simulink model "xytheta_microcontroller"  (R2022a)
settings: Solver=VariableStepAuto  StartTime=0.0  StopTime=stop_time  RelTol=1e-3
values from neighbouring files (symbols this model uses):
  a1 = [0.0226481432906 0.0228584411445 0.0225295964484 0.0217518027828 0.0203868263557 0.0184221135046 0.0156410240283 0.0121230277389 0.00798950755081 0.00344770073943 -0.00140524350521 -0.00605971322152 ... (2997 elements, 37x9x9)]    [femm_output.mat]    (also in hi.mat = [0.040259405186 0.0403013496491 0.0403539168343 0.0403184727; test.mat = [0.0334886294169 0.0187353722544 -0.0188188604787 -0.0334886)
  a2 = [0.0289816801878 0.0282562064819 0.0268804805083 0.0249372347426 0.0221345937075 0.0184340302923 0.0137477378532 0.00803353156156 0.0017047126462 -0.0048350371899 -0.0110157154995 -0.01647453575 ... (2997 elements, 37x9x9)]    [femm_output.mat]    (also in hi.mat = [0.0510882717013 0.051015840912 0.0508647790068 0.0507223197; test.mat = [0.0338593341727 0.0189905412856 -0.0197522315336 -0.0338593)
  a3 = [0.0115535270098 0.0148029062382 0.0173877315644 0.0193612077509 0.0206442979737 0.0215000532697 0.021876503755 0.0217878376451 0.0212671436174 0.0202424961232 0.0185927416037 0.0163372080044 ... (2997 elements, 37x9x9)]    [femm_output.mat]    (also in hi.mat = [0.0214255858237 0.0226377892342 0.0238084550149 0.024930652; test.mat = [0.0190432080829 0.0343100490551 0.0190529625979 -0.01904320)
  a4 = [0.0199201516492 0.0239463634306 0.0268101507336 0.0287527989045 0.0300172301517 0.0306310326126 0.0306116684575 0.0301535034256 0.0292209899207 0.0275296444333 0.0250546319784 0.0217006548338 ... (2997 elements, 37x9x9)]    [femm_output.mat]    (also in hi.mat = [0.0351552019156 0.0366796893809 0.0381457834123 0.039508739; test.mat = [0.0191793003104 0.0345170149993 0.0192239303836 -0.01917930)
  b1 = [-0.0198768129153 -0.0149244319576 -0.00858526905599 -0.00187364461528 0.0050977168348 0.0114478894775 0.0171037743603 0.0216638634405 0.0251231705896 0.0275944419023 0.0292021825363 0.0301941032583 ... (2997 elements, 37x9x9)]    [femm_output.mat]    (also in hi.mat = [-0.0351292809325 -0.0335210392107 -0.0318149846307 -0.03001; test.mat = [-0.0195035950206 0.0204454837762 0.032908216348 0.019503595)
  b2 = [-0.0115479896023 -0.00770288201737 -0.00341093185035 0.0012077259201 0.00577057398931 0.00982413393911 0.0134313300768 0.0163555375406 0.0185311126654 0.0202513667265 0.0212470983786 0.0217997189875 ... (2997 elements, 37x9x9)]    [femm_output.mat]    (also in hi.mat = [-0.0214309796469 -0.0201513971109 -0.018842107593 -0.017472; test.mat = [-0.0191855417866 0.0192130384034 0.0341712245421 0.01918554)
  b3 = [-0.0290438679046 -0.0293208138251 -0.0289621611228 -0.0282127308736 -0.0266510102895 -0.0242723997603 -0.0209097969042 -0.0164709315768 -0.011084328795 -0.00477482143157 0.00165462601804 0.00800924150907 ... (2997 elements, 37x9x9)]    [femm_output.mat]    (also in hi.mat = [-0.0511327637629 -0.0511785516059 -0.0512008658749 -0.05117; test.mat = [-0.0346544389103 -0.0187806132998 0.0188182643543 0.0346544)
  b4 = [-0.0226529885689 -0.0220487060527 -0.0209138863789 -0.0192567684963 -0.016982348983 -0.0139643562445 -0.0103025939746 -0.00604882885267 -0.00143455513257 0.00343618932918 0.00801414292928 0.012190086562 ... (2997 elements, 37x9x9)]    [femm_output.mat]    (also in hi.mat = [-0.0402522375725 -0.0401755201934 -0.0400474470218 -0.03988; test.mat = [-0.033778561725 -0.0189587155081 0.0201521885325 0.03377856)
  c1 = [-0.018042933605 -0.0207358233247 -0.0226807589747 -0.0238865774927 -0.0245474910314 -0.0246583171435 -0.0242673887984 -0.0234585855422 -0.0221202260013 -0.0200782518148 -0.017518348181 -0.0141731707546 ... (2997 elements, 37x9x9)]    [femm_output.mat]    (also in hi.mat = [-0.0297253197394 -0.0308627231265 -0.0319523431791 -0.03294; test.mat = [-0.0182900065298 -0.0340093058074 -0.0190263778387 0.018290)
  c2 = [-0.0111046794327 -0.0156541395447 -0.0193854693358 -0.0221379319248 -0.0242137197455 -0.0256527501849 -0.0265983628578 -0.0270163619409 -0.0268882455917 -0.0262763125893 -0.0249792360852 -0.0229784347415 ... (2997 elements, 37x9x9)]    [femm_output.mat]    (also in hi.mat = [-0.0234193013701 -0.0250617295759 -0.0266424676889 -0.02819; test.mat = [-0.0188563417261 -0.033847126142 -0.0190525067235 0.0188563)
  c3 = [0.0110989874251 0.00587027765918 4.48039996108e-05 -0.00583886766056 -0.0113087799728 -0.0160948615017 -0.0199647800731 -0.0229326844268 -0.0249385554175 -0.0262624574827 -0.0268970230309 -0.0270019496976 ... (2997 elements, 37x9x9)]    [femm_output.mat]    (also in hi.mat = [0.0233910963939 0.0216737015426 0.0198604309257 0.018009200; test.mat = [0.0190983781671 -0.0185938316594 -0.0330743417046 -0.019098)
  c4 = [0.0180276596334 0.0143851403822 0.0100683328735 0.00515693164411 -8.40566002638e-05 -0.00533297487089 -0.0100594562482 -0.0142052505478 -0.017542507454 -0.0201282699008 -0.0221308552047 -0.0234805966963 ... (2997 elements, 37x9x9)]    [femm_output.mat]    (also in hi.mat = [0.0297436396273 0.0285474856426 0.0272933586912 0.025981890; test.mat = [0.0190714466776 -0.0196627612069 -0.0337734384564 -0.019071)
  theta_r_in = [0 5 10 15 20 25 30 35 40 45 50 55 ... (37 elements, 1x37)]    [femm_output.mat]    (also in hi.mat = [0 1 2 3 4 5 6 7 8 9 10 11 ... (180 elements, 1x180)]; test.mat = [0 30 60 90 120 150])
  x_position = [-2 -1.5 -1 -0.5 0 0.5 1 1.5 2]    [femm_output.mat]    (also in hi.mat; test.mat = 0)
  y_position = [-2 -1.5 -1 -0.5 0 0.5 1 1.5 2]    [femm_output.mat]    (also in hi.mat; test.mat = 0)
undefined symbols (not defined in the file or in its folder): fs_theta, x_sampletime, y_sampletime
libraries: dspsrcs4 x3, simulink x1
settings Model: Creator=qorgud1209  LastModifiedBy=baikhyeongmeon
settings DebuggingCC: UnconnectedInputMsg=warning  UnconnectedOutputMsg=warning  UnconnectedLineMsg=warning
settings SFSimCC: SimCustomHeaderCode="#include \"microcontroller.h\""  SimUserSources=microcontroller.c  SimAnalyzeCustomCode=on  CustomCodeGlobalsAsFunctionIO=on
settings RTWCC: DLArmComputeVersion=19.05

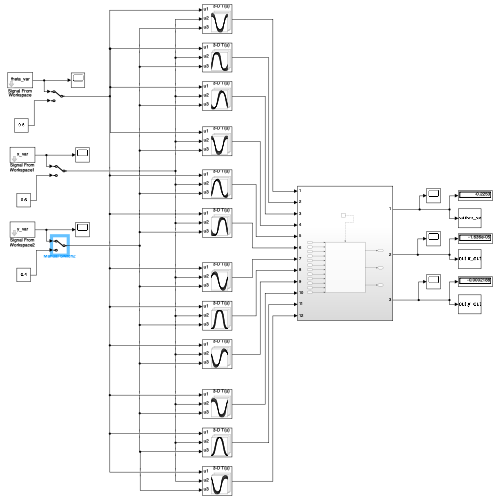
[thumbnail: Simulink's stored preview of the top-level diagram]
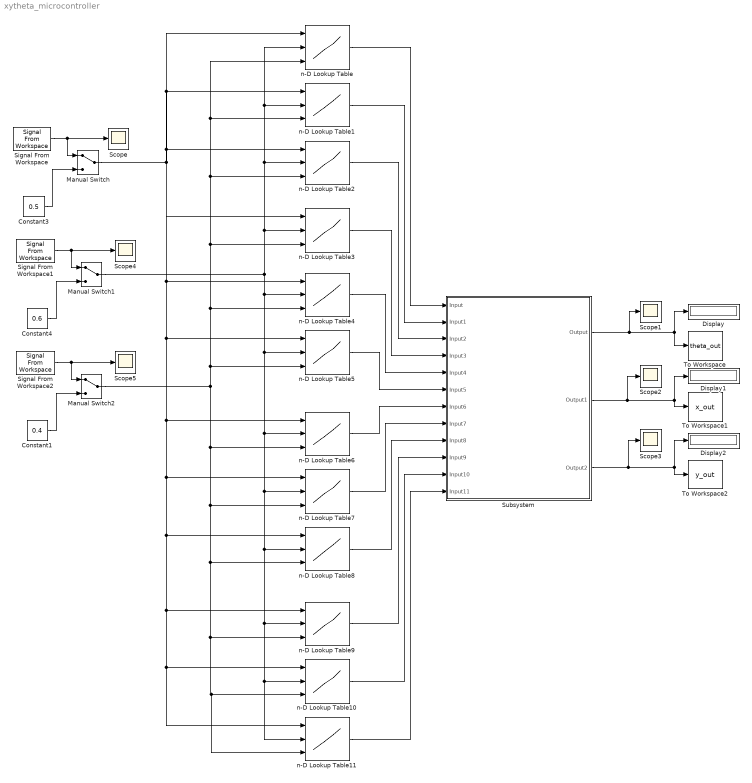
== system xytheta_microcontroller ==
  Constant1 : Constant  Value=0.4
  Constant3 : Constant  Value=0.5
  Constant4 : Constant  Value=0.6
  Display : Display
  Display1 : Display
  Display2 : Display
  Manual Switch : ManualSwitch
  Manual Switch1 : ManualSwitch
  Manual Switch2 : ManualSwitch
  Scope{,1..5} (6 alike) : Scope
  Signal From Workspace : dspsrcs4/Signal From Workspace  X=theta_var  Ts=1/fs_theta  nsamps=numframe_theta  OutputAfterFinalValue=Setting to zero  ignoreOrWarnInputAndFrameLengths=off  OutputFrames=off
  Signal From Workspace1 : dspsrcs4/Signal From Workspace  X=x_var  Ts=x_sampletime  nsamps=1  OutputAfterFinalValue=Setting to zero  ignoreOrWarnInputAndFrameLengths=off  OutputFrames=off
  Signal From Workspace2 : dspsrcs4/Signal From Workspace  X=y_var  Ts=y_sampletime  nsamps=1  OutputAfterFinalValue=Setting to zero  ignoreOrWarnInputAndFrameLengths=off  OutputFrames=off
  Subsystem : Subsystem
  To Workspace : ToWorkspace  VariableName=theta_out  SampleTime=-1
      settings: Save2DSignal=2-D array (concatenate along first dimension)
  To Workspace1 : ToWorkspace  VariableName=x_out  SampleTime=-1
      settings: Save2DSignal=2-D array (concatenate along first dimension)
  To Workspace2 : ToWorkspace  VariableName=y_out  SampleTime=-1
      settings: Save2DSignal=2-D array (concatenate along first dimension)
  n-D Lookup Table : Lookup_n-D  NumberOfTableDimensions=3  BreakpointsForDimension1=theta_r_in  BreakpointsForDimension2=x_position  BreakpointsForDimension3=y_position  Table=a1  InternalRulePriority=Speed  RndMeth=Simplest
      settings: InputPortMap=u0,u1,u2
  n-D Lookup Table1 : Lookup_n-D  NumberOfTableDimensions=3  BreakpointsForDimension1=theta_r_in  BreakpointsForDimension2=x_position  BreakpointsForDimension3=y_position  Table=b1  InternalRulePriority=Speed  RndMeth=Simplest
      settings: InputPortMap=u0,u1,u2
  n-D Lookup Table10 : Lookup_n-D  NumberOfTableDimensions=3  BreakpointsForDimension1=theta_r_in  BreakpointsForDimension2=x_position  BreakpointsForDimension3=y_position  Table=b4  InternalRulePriority=Speed  RndMeth=Simplest
      settings: InputPortMap=u0,u1,u2
  n-D Lookup Table11 : Lookup_n-D  NumberOfTableDimensions=3  BreakpointsForDimension1=theta_r_in  BreakpointsForDimension2=x_position  BreakpointsForDimension3=y_position  Table=c4  InternalRulePriority=Speed  RndMeth=Simplest
      settings: InputPortMap=u0,u1,u2
  n-D Lookup Table2 : Lookup_n-D  NumberOfTableDimensions=3  BreakpointsForDimension1=theta_r_in  BreakpointsForDimension2=x_position  BreakpointsForDimension3=y_position  Table=c1  InternalRulePriority=Speed  RndMeth=Simplest
      settings: InputPortMap=u0,u1,u2
  n-D Lookup Table3 : Lookup_n-D  NumberOfTableDimensions=3  BreakpointsForDimension1=theta_r_in  BreakpointsForDimension2=x_position  BreakpointsForDimension3=y_position  Table=a2  InternalRulePriority=Speed  RndMeth=Simplest
      settings: InputPortMap=u0,u1,u2
  n-D Lookup Table4 : Lookup_n-D  NumberOfTableDimensions=3  BreakpointsForDimension1=theta_r_in  BreakpointsForDimension2=x_position  BreakpointsForDimension3=y_position  Table=b2  InternalRulePriority=Speed  RndMeth=Simplest
      settings: InputPortMap=u0,u1,u2
  n-D Lookup Table5 : Lookup_n-D  NumberOfTableDimensions=3  BreakpointsForDimension1=theta_r_in  BreakpointsForDimension2=x_position  BreakpointsForDimension3=y_position  Table=c2  InternalRulePriority=Speed  RndMeth=Simplest
      settings: InputPortMap=u0,u1,u2
  n-D Lookup Table6 : Lookup_n-D  NumberOfTableDimensions=3  BreakpointsForDimension1=theta_r_in  BreakpointsForDimension2=x_position  BreakpointsForDimension3=y_position  Table=a3  InternalRulePriority=Speed  RndMeth=Simplest
      settings: InputPortMap=u0,u1,u2
  n-D Lookup Table7 : Lookup_n-D  NumberOfTableDimensions=3  BreakpointsForDimension1=theta_r_in  BreakpointsForDimension2=x_position  BreakpointsForDimension3=y_position  Table=b3  InternalRulePriority=Speed  RndMeth=Simplest
      settings: InputPortMap=u0,u1,u2
  n-D Lookup Table8 : Lookup_n-D  NumberOfTableDimensions=3  BreakpointsForDimension1=theta_r_in  BreakpointsForDimension2=x_position  BreakpointsForDimension3=y_position  Table=c3  InternalRulePriority=Speed  RndMeth=Simplest
      settings: InputPortMap=u0,u1,u2
  n-D Lookup Table9 : Lookup_n-D  NumberOfTableDimensions=3  BreakpointsForDimension1=theta_r_in  BreakpointsForDimension2=x_position  BreakpointsForDimension3=y_position  Table=a4  InternalRulePriority=Speed  RndMeth=Simplest
      settings: InputPortMap=u0,u1,u2
  wires:
  Manual Switch/1 -> n-D Lookup Table11/1, n-D Lookup Table10/1, n-D Lookup Table9/1, n-D Lookup Table8/1, n-D Lookup Table7/1, n-D Lookup Table6/1, n-D Lookup Table5/1, n-D Lookup Table4/1, n-D Lookup Table/1, n-D Lookup Table1/1, n-D Lookup Table3/1, n-D Lookup Table2/1
  Manual Switch2/1 -> n-D Lookup Table4/3, n-D Lookup Table3/3, n-D Lookup Table1/3, n-D Lookup Table/3, n-D Lookup Table2/3, n-D Lookup Table5/3, n-D Lookup Table6/3, n-D Lookup Table7/3, n-D Lookup Table8/3, n-D Lookup Table11/3, n-D Lookup Table10/3, n-D Lookup Table9/3
  Manual Switch1/1 -> n-D Lookup Table3/2, n-D Lookup Table1/2, n-D Lookup Table/2, n-D Lookup Table2/2, n-D Lookup Table4/2, n-D Lookup Table6/2, n-D Lookup Table9/2, n-D Lookup Table11/2, n-D Lookup Table10/2, n-D Lookup Table8/2, n-D Lookup Table7/2, n-D Lookup Table5/2
  n-D Lookup Table/1 -> Subsystem/1(Input)
  n-D Lookup Table1/1 -> Subsystem/2(Input1)
  Subsystem/1(Output) -> Scope1/1, To Workspace/1, Display/1
  Subsystem/2(Output1) -> Scope2/1, To Workspace1/1, Display1/1
  n-D Lookup Table2/1 -> Subsystem/3(Input2)
  n-D Lookup Table3/1 -> Subsystem/4(Input3)
  n-D Lookup Table4/1 -> Subsystem/5(Input4)
  n-D Lookup Table5/1 -> Subsystem/6(Input5)
  n-D Lookup Table6/1 -> Subsystem/7(Input6)
  n-D Lookup Table7/1 -> Subsystem/8(Input7)
  n-D Lookup Table8/1 -> Subsystem/9(Input8)
  n-D Lookup Table9/1 -> Subsystem/10(Input9)
  n-D Lookup Table10/1 -> Subsystem/11(Input10)
  n-D Lookup Table11/1 -> Subsystem/12(Input11)
  Signal From Workspace/1 -> Manual Switch/1, Scope/1
  Constant3/1 -> Manual Switch/2
  Subsystem/3(Output2) -> Scope3/1, To Workspace2/1, Display2/1
  Signal From Workspace1/1 -> Scope4/1, Manual Switch1/1
  Constant4/1 -> Manual Switch1/2
  Signal From Workspace2/1 -> Scope5/1, Manual Switch2/1
  Constant1/1 -> Manual Switch2/2

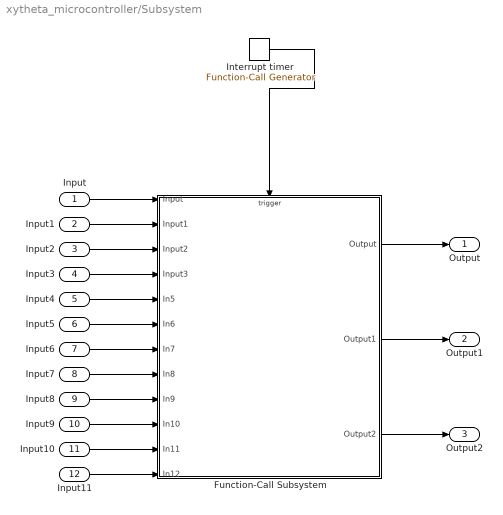
== system xytheta_microcontroller/Subsystem ==
  Input : Inport
  Input1 : Inport  Port=2
  Input2 : Inport  Port=3
  Input3 : Inport  Port=4
  Input4 : Inport  Port=5
  Input5 : Inport  Port=6
  Input6 : Inport  Port=7
  Input7 : Inport  Port=8
  Input8 : Inport  Port=9
  Input9 : Inport  Port=10
  Input10 : Inport  Port=11
  Input11 : Inport  Port=12
  Function-Call Subsystem : Subsystem  TreatAsAtomicUnit=on
  Interrupt timer : simulink/Ports & Subsystems/Function-Call Generator  sample_time=Ts  numberOfIterations=1  DisallowWideOutput=off
  Output : Outport
  Output1 : Outport  Port=2
  Output2 : Outport  Port=3
  wires:
  Interrupt timer/1 -> Function-Call Subsystem/Trigger
  Input/1 -> Function-Call Subsystem/1(Input)
  Input1/1 -> Function-Call Subsystem/2(Input1)
  Input2/1 -> Function-Call Subsystem/3(Input2)
  Input3/1 -> Function-Call Subsystem/4(Input3)
  Input5/1 -> Function-Call Subsystem/6(In6)
  Input4/1 -> Function-Call Subsystem/5(In5)
  Input6/1 -> Function-Call Subsystem/7(In7)
  Input7/1 -> Function-Call Subsystem/8(In8)
  Input9/1 -> Function-Call Subsystem/10(In10)
  Input8/1 -> Function-Call Subsystem/9(In9)
  Input10/1 -> Function-Call Subsystem/11(In11)
  Input11/1 -> Function-Call Subsystem/12(In12)
  Function-Call Subsystem/1(Output) -> Output/1
  Function-Call Subsystem/2(Output1) -> Output1/1
  Function-Call Subsystem/3(Output2) -> Output2/1

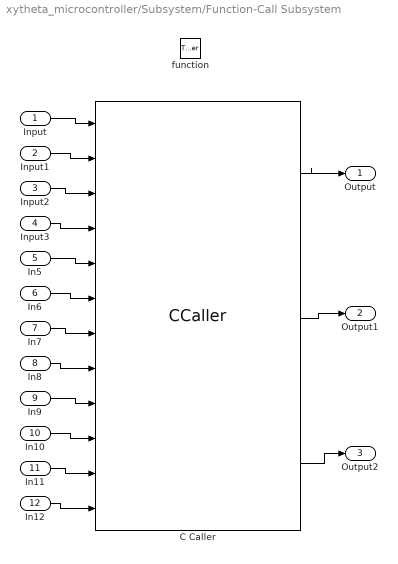
== system xytheta_microcontroller/Subsystem/Function-Call Subsystem ==
  Input : Inport
  Input1 : Inport  Port=2
  Input2 : Inport  Port=3
  Input3 : Inport  Port=4
  In5 : Inport  Port=5
  In6 : Inport  Port=6
  In7 : Inport  Port=7
  In8 : Inport  Port=8
  In9 : Inport  Port=9
  In10 : Inport  Port=10
  In11 : Inport  Port=11
  In12 : Inport  Port=12
  function : TriggerPort  TriggerType=function-call  VariantControl=(inherit)
  C Caller : CCaller  FunctionName=microcontroller  PortSpecificationStruct="%)30     .    \"!D   8    (     @         %    \"     \\    !     0         %  0 \"0    $    _    07)G3F%M90  4&]R=$YA;64 4V-O<&4     26YD97@     5'EP90      4VEZ90      27-';&]B86P   X    P    !@    @    $          4    (     0    0    !         !  ! !A9&,Q#@   #     &    \"     0         !0    @    !    !     $         $  $ &%D8S$.    .     8    (    !          %    \"     $    %     0         0 ...(+8273 chars)"
  Output : Outport  OutDataTypeStr=double
  Output1 : Outport  Port=2  OutDataTypeStr=double
  Output2 : Outport  Port=3  OutDataTypeStr=double
  wires:
  Input/1 -> C Caller/1
  Input1/1 -> C Caller/2
  Input2/1 -> C Caller/3
  In6/1 -> C Caller/6
  In5/1 -> C Caller/5
  Input3/1 -> C Caller/4
  In7/1 -> C Caller/7
  In8/1 -> C Caller/8
  In9/1 -> C Caller/9
  In10/1 -> C Caller/10
  In11/1 -> C Caller/11
  In12/1 -> C Caller/12
  C Caller/1 -> Output/1
  C Caller/2 -> Output1/1
  C Caller/3 -> Output2/1
